simulink model "anti_condensation_control"  (R2025a)
settings: Solver=FixedStepDiscrete  StartTime=0.0  StopTime=5400  FixedStep=0.5  RelTol=1e-3
StopFcn:
  | try
  |     so = evalin('base', 'simOut');
  |     T_amb = so.get('T_amb_out').Data(:);
  |     T_ctrl = so.get('T_mod_out').Data(:);
  |     T_nc   = so.get('T_mod_nc_out').Data(:);
  | catch
  |     if ~exist('T_amb_out','var') || ~exist('T_mod_out','var') || ~exist('T_mod_nc_out','var'); return; end
  |     T_amb = T_amb_out(:); T_ctrl = T_mod_out(:); T_nc = T_mod_nc_out(:);
  | end
  | dt = 0.5; dT_threshold = 5; dT_second = 7;
  | n = min([length(T_ctrl), length(T_nc), length(T_amb)]);
  | t_min = (0:dt:(n-1)*dt)' / 60;
  | T_ctrl = T_ctrl(1:n); T_nc = T_nc(1:n); T_amb = T_amb(1:n);
  | dT_ctrl = T_amb - T_ctrl; dT_nc = T_amb - T_nc;
  | in_risk_ctrl = dT_ctrl > dT_threshold; in_risk_nc = dT_nc > dT_threshold;
  | risk_dur_ctrl = sum(in_risk_ctrl)*dt/60; risk_dur_nc = sum(in_risk_nc)*dt/60;
  | peak_ctrl = max(dT_ctrl); peak_nc = max(dT_nc);
  | exp_ctrl = sum(max(dT_ctrl-dT_threshold,0))*dt/60; exp_nc = sum(max(dT_nc-dT_threshold,0))*dt/60;
  | 
  | % --- 绘图 ---
  | set(groot,'DefaultFigureColor','w','DefaultAxesColor','w');
  | figure('Name','防凝露控制效果对比 - Simulink仿真','Position',[100 100 1400 500],'Color','w');
  | 
  | subplot(1,4,1); plot(t_min,T_ctrl,'b-','LineWidth',1.8); hold on;
  | plot(t_min,T_nc,'r--','LineWidth',1.5); plot(t_min,T_amb,'k:','LineWidth',1);
  | xlabel('时间 (min)'); ylabel('温度 (°C)'); title('模块温度对比');
  | legend('有控制','无控制','环境','Location','best'); grid on;
  | 
  | subplot(1,4,2); plot(t_min,dT_ctrl,'b-','LineWidth',1.8); hold on;
  | plot(t_min,dT_nc,'r--','LineWidth',1.5); yline(dT_threshold,'k--','凝露阈值','LineWidth',1.5);
  | xlabel('时间 (min)'); ylabel('\Delta T = T_{amb} - T_{mod} (°C)'); title('温差对比 (全程)');
  | legend('有控制','无控制','Location','best'); grid on;
  | 
  | subplot(1,4,3); idx20=find(t_min<=20);
  | plot(t_min(idx20),dT_ctrl(idx20),'b-','LineWidth',1.8); hold on;
  | plot(t_min(idx20),dT_nc(idx20),'r--','LineWidth',1.5);
  | yline(dT_threshold,'k--','凝露阈值','LineWidth',1.5);
  | yline(dT_second,'m:','第二温差','LineWidth',1);
  | xlabel('时间 (min)'); ylabel('\Delta T (°C)'); title('前20分钟瞬态放大');
  | legend('有控制','无控制','Location','best'); grid on;
  | 
  | subplot(1,4,4); bar_data=[risk_dur_ctrl risk_dur_nc; peak_ctrl peak_nc; exp_ctrl exp_nc]';
  | b=bar(bar_data); b(1).FaceColor='b'; b(2).FaceColor='r';
  | set(gca,'XTickLabel',{'风险时长(min)','峰值温差(°C)','暴露量(°C·min)'});
  | legend('有控制','无控制','Location','northwest');
  | title('防凝露效果对比'); ylabel('指标值'); grid on;
  | 
  | sgtitle('防凝露控制效果对比 - Simulink 模型仿真 (专利 CN 121984334 A)');
  | 
  | % --- 控制台输出 ---
  | disp(' ');
  | disp('===== 风险指标 (Simulink自动输出) =====');
  | disp(['风险时长: ' num2str(risk_dur_ctrl,'%.1f') ' min (有控制) vs ' num2str(risk_dur_nc,'%.1f') ' min (无控制) -> 缩短 ' num2str((risk_dur_nc-risk_dur_ctrl)/risk_dur_nc*100,'%.1f') '%']);
  | disp(['峰值温差: ' num2str(peak_ctrl,'%.2f') ' degC (有控制) vs ' num2str(peak_nc,'%.2f') ' degC (无控制) -> 降低 ' num2str((peak_nc-peak_ctrl)/peak_nc*100,'%.1f') '%']);
  | disp(['暴露量:   ' num2str(exp_ctrl,'%.1f') ' degC*min (有控制) vs ' num2str(exp_nc,'%.1f') ' degC*min (无控制) -> 减少 ' num2str((exp_nc-exp_ctrl)/exp_nc*100,'%.1f') '%']);
  | 
  | % --- 保存图片 ---
  | scriptDir = fileparts(which('anti_condensation_control'));
  | if ~isempty(scriptDir)
  |     saveas(gcf, fullfile(scriptDir, 'simulink_comparison.png'));
  |     disp('对比图已自动保存: simulink_comparison.png');
  | end
model workspace (MAT data in the model file):
  C_th = 1000
  P_loss0 = 12
  R_th0 = 0.48
  T_mod0 = 27
  V_max = 880
  V_min = 580
  V_nom = 620
  dT_2nd = 7
  dT_first = 4
  dT_th = 5
  dV_step = 40
  dt = 0.5
  fan_min = 50
  fan_nom = 100
undefined symbols (not defined in the file or in its folder): DiscIntNeverNeededParam, dspblkCoreblockFVToolHelper, gcbh
settings Model: Creator=jicai  LastModifiedBy=jicai
settings DataIOCC: ReturnWorkspaceOutputsName=simOut

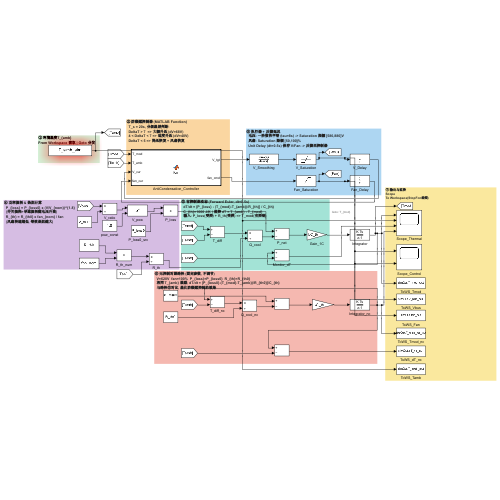
[thumbnail: Simulink's stored preview of the top-level diagram]
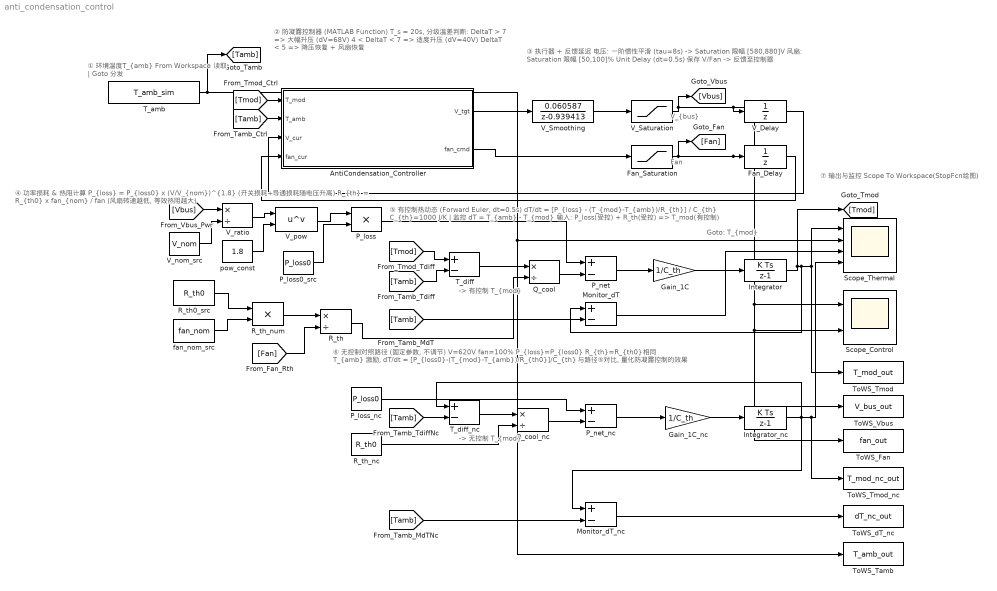
== system anti_condensation_control ==
  note: ① 环境温度T_{amb}
      | From Workspace 读取 | Goto 分发
  note: ② 防凝露控制器 (MATLAB Function)
      |   T_s = 20s, 分级温差判断:
      |   DeltaT > 7  => 大幅升压 (dV=68V)
      |   4 < DeltaT < 7 => 适度升压 (dV=40V)
      |   DeltaT < 5 => 降压恢复 + 风扇恢复
  note: ③ 执行器 + 反馈延迟
      |   电压: 一阶惯性平滑 (tau=8s) -> Saturation 限幅 [580,880]V
      |   风扇: Saturation 限幅 [50,100]%
      |   Unit Delay (dt=0.5s) 保存 V/Fan -> 反馈至控制器
  note: ④ 功率损耗 & 热阻计算
      |   P_{loss} = P_{loss0} x (V/V_{nom})^{1.8}
      |   (开关损耗+导通损耗随电压升高)
      |   R_{th} = R_{th0} x fan_{nom} / fan
      |   (风扇转速越低, 等效热阻越大)
  note: ⑤ 有控制热动态 (Forward Euler, dt=0.5s)
      |   dT/dt = [P_{loss} - (T_{mod}-T_{amb})/R_{th}] / C_{th}
      |   C_{th}=1000 J/K | 监控 dT = T_{amb} - T_{mod}
      |   输入: P_loss(受控) + R_th(受控) => T_mod(有控制)
  note: ⑥ 无控制对照路径 (固定参数, 不调节)
      |   V=620V  fan=100%  P_{loss}=P_{loss0}  R_{th}=R_{th0}
      |   相同 T_{amb} 激励, dT/dt = [P_{loss0}-(T_{mod}-T_{amb})/R_{th0}]/C_{th}
      |   与路径⑤对比, 量化防凝露控制的效果
  note: ⑦ 输出与监控
      | Scope
      | To Workspace(StopFcn绘图)
  note: Goto: T_{mod}
  note: V_{bus}
  note: Fan
  note: -> 有控制 T_{mod}
  note: -> 无控制 T_{mod}
  AntiCondensation_Controller : MATLAB Function  TreatAsAtomicUnit=on
  Fan_Delay : UnitDelay  InitialCondition=100  SampleTime=0.5  HasFrameUpgradeWarning=on
  Fan_Saturation : Saturate  UpperLimit=100  LowerLimit=fan_min
  Gain_1C : Gain  Gain=1/C_th
  Gain_1C_nc : Gain  Gain=1/C_th
  Integrator : DiscreteIntegrator  InitialCondition=T_mod0  SampleTime=0.5  ICPrevOutput=DiscIntNeverNeededParam  ICPrevScaledInput=DiscIntNeverNeededParam
  Integrator_nc : DiscreteIntegrator  InitialCondition=T_mod0  SampleTime=0.5  ICPrevOutput=DiscIntNeverNeededParam  ICPrevScaledInput=DiscIntNeverNeededParam
  Monitor_dT : Sum  Inputs=+-
  Monitor_dT_nc : Sum  Inputs=+-
  P_loss : Product  Inputs=**
  P_loss0_src : Constant  Value=P_loss0
  P_loss_nc : Constant  Value=P_loss0
  P_net : Sum  Inputs=+-
  P_net_nc : Sum  Inputs=+-
  Q_cool : Product  Inputs=*/
  Q_cool_nc : Product  Inputs=*/
  R_th : Product  Inputs=*/
  R_th0_src : Constant  Value=R_th0
  R_th_nc : Constant  Value=R_th0
  R_th_num : Product  Inputs=**
  Scope_Control : Scope  NumInputPorts=2
  Scope_Thermal : Scope  NumInputPorts=4
  T_amb : FromWorkspace  VariableName=T_amb_sim  SampleTime=0.5
  T_diff : Sum  Inputs=+-
  T_diff_nc : Sum  Inputs=+-
  ToWS_Fan : ToWorkspace  VariableName=fan_out  SaveFormat=Timeseries  SampleTime=-1
  ToWS_Tamb : ToWorkspace  VariableName=T_amb_out  SaveFormat=Timeseries  SampleTime=-1
  ToWS_Tmod : ToWorkspace  VariableName=T_mod_out  SaveFormat=Timeseries  SampleTime=-1
  ToWS_Tmod_nc : ToWorkspace  VariableName=T_mod_nc_out  SaveFormat=Timeseries  SampleTime=-1
  ToWS_Vbus : ToWorkspace  VariableName=V_bus_out  SaveFormat=Timeseries  SampleTime=-1
  ToWS_dT_nc : ToWorkspace  VariableName=dT_nc_out  SaveFormat=Timeseries  SampleTime=-1
  V_Delay : UnitDelay  InitialCondition=620  SampleTime=0.5  HasFrameUpgradeWarning=on
  V_Saturation : Saturate  UpperLimit=V_max  LowerLimit=V_min
  V_Smoothing : DiscreteTransferFcn  LoadFcn=dspblkCoreblockFVToolHelper(gcbh,'load');  Numerator=0.060587  Denominator=[1, -0.939413]  InitialStates=620  SampleTime=0.5
      settings: CopyFcn=dspblkCoreblockFVToolHelper(gcbh,'copy');  DeleteFcn=dspblkCoreblockFVToolHelper(gcbh,'close');  ModelCloseFcn=dspblkCoreblockFVToolHelper(gcbh,'close');  PreSaveFcn=dspblkCoreblockFVToolHelper(gcbh,'presave');  PostSaveFcn=dspblkCoreblockFVToolHelper(gcbh,'postsave');  CloseFcn=dspblkCoreblockFVToolHelper(gcbh,'close');
  V_nom_src : Constant  Value=V_nom
  V_pow : Math  Operator=pow
  V_ratio : Product  Inputs=*/
  fan_nom_src : Constant  Value=fan_nom
  pow_const : Constant  Value=1.8
  wires:
  T_amb/1 -> Scope_Thermal/2, ToWS_Tamb/1, [Tamb]
  [Tamb] -> AntiCondensation_Controller/2(T_amb)
  [Tamb] -> T_diff/2
  [Tamb] -> Monitor_dT/2
  [Tamb] -> T_diff_nc/2
  [Tamb] -> Monitor_dT_nc/2
  Integrator/1 -> Scope_Thermal/1, ToWS_Tmod/1, Monitor_dT/1, [Tmod]
  [Tmod] -> AntiCondensation_Controller/1(T_mod)
  [Tmod] -> T_diff/1
  V_Delay/1 -> AntiCondensation_Controller/3(V_cur)
  Fan_Delay/1 -> AntiCondensation_Controller/4(fan_cur)
  AntiCondensation_Controller/1(V_tgt) -> V_Smoothing/1
  V_Smoothing/1 -> V_Saturation/1
  AntiCondensation_Controller/2(fan_cmd) -> Fan_Saturation/1
  V_Saturation/1 -> Scope_Control/1, ToWS_Vbus/1, V_Delay/1, [Vbus]
  Fan_Saturation/1 -> Scope_Control/2, ToWS_Fan/1, Fan_Delay/1, [Fan]
  [Vbus] -> V_ratio/1
  V_nom_src/1 -> V_ratio/2
  V_ratio/1 -> V_pow/1
  pow_const/1 -> V_pow/2
  V_pow/1 -> P_loss/1
  P_loss0_src/1 -> P_loss/2
  R_th0_src/1 -> R_th_num/1
  fan_nom_src/1 -> R_th_num/2
  R_th_num/1 -> R_th/1
  [Fan] -> R_th/2
  T_diff/1 -> Q_cool/1
  R_th/1 -> Q_cool/2
  P_loss/1 -> P_net/1
  Q_cool/1 -> P_net/2
  P_net/1 -> Gain_1C/1
  Gain_1C/1 -> Integrator/1
  Integrator_nc/1 -> Monitor_dT_nc/1, T_diff_nc/1, Scope_Thermal/4, ToWS_Tmod_nc/1
  T_diff_nc/1 -> Q_cool_nc/1
  R_th_nc/1 -> Q_cool_nc/2
  P_loss_nc/1 -> P_net_nc/1
  Q_cool_nc/1 -> P_net_nc/2
  P_net_nc/1 -> Gain_1C_nc/1
  Gain_1C_nc/1 -> Integrator_nc/1
  Monitor_dT/1 -> Scope_Thermal/3
  Monitor_dT_nc/1 -> ToWS_dT_nc/1

== matlab function anti_condensation_control/AntiCondensation_Controller ==
  data: T_mod input; V_tgt output; T_amb input; V_cur input; fan_cur input; fan_cmd output
function [V_tgt, fan_cmd] = fcn(T_mod, T_amb, V_cur, fan_cur)
%#codegen
persistent tick
persistent V_target
if isempty(tick)
    tick = 0;
    V_target = 620.0;
end
deltaT = T_amb - T_mod;
fan_cmd = fan_cur;
if tick == 0
    if deltaT > 5.0
        if deltaT > 7.0
            V_target = min(V_cur + 68.0, 880);
        elseif deltaT > 4.0
            V_target = min(V_cur + 40, 880);
        end
    else
        if V_cur > 625.0
            V_target = max(620.0, V_cur - 24.0);
        end
        if V_cur > 700.0
            fan_cmd = max(fan_cur - 6.0, 50);
        end
        if fan_cur < 97.0 && V_cur <= 630.0
            fan_cmd = min(100.0, fan_cur + 5.0);
        end
    end
end
tick = tick + 1;
if tick >= 40
    tick = 0;
end
V_tgt = V_target;
end
